simulink model "A02_L9_0"  (R2016b)
settings: Solver=ode45  StartTime=0.0  StopTime=40.0  RelTol=1e-3  EnableMultiTasking=on
settings Model: Creator=User  LastModifiedBy=mluser
settings DataIOCC: LimitDataPoints=on  SaveFormat=Array
settings OptimizationCC: LifeSpan=inf
settings DebuggingCC: SolverPrmCheckMsg=warning  SFUnexpectedBacktrackingDiag=warning  SFNoUnconditionalDefaultTransitionDiag=warning  SFExecutionAtInitializationDiag=none
settings HardwareCC: ProdBitPerPointer=32  ProdBitPerSizeT=32  ProdBitPerPtrDiffT=32  ProdLargestAtomicFloat=None  ProdIntDivRoundTo=Undefined  ProdEndianess=Unspecified  ProdWordSize=32  ProdHWDeviceType=32-bit Generic
settings ModelReferenceCC: PropagateSignalLabelsOutOfModel=off
settings GRTTargetCC: TargetLangStandard=C89/C90 (ANSI)
settings ConfigComp: CovMetricSettings=dw  CovSaveCumulativeToWorkspaceVar=on  CovSaveSingleToWorkspaceVar=on  CovExternalEMLEnable=off  CovSFcnEnable=off

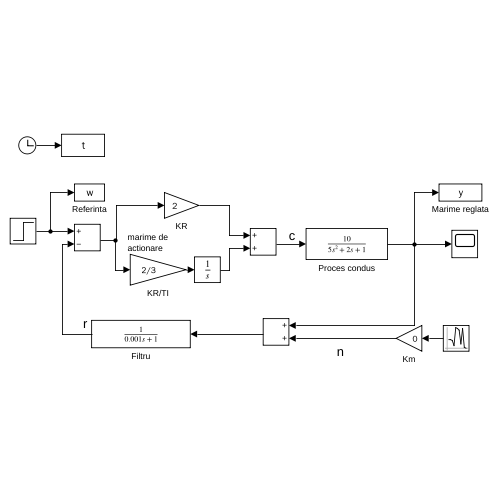
[thumbnail: Simulink's stored preview of the top-level diagram]
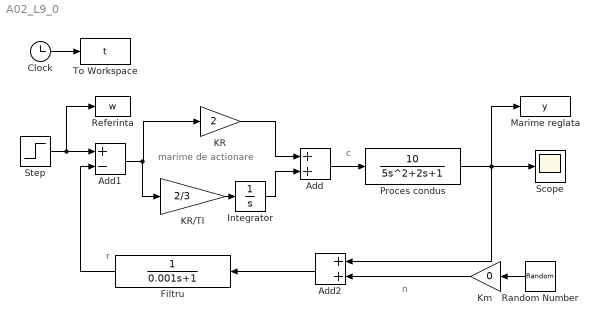
== system A02_L9_0 ==
  note: n
  note: r
  note: c
  note: marime de
      | actionare
  Add : Sum
  Add1 : Sum  Inputs=+-
  Add2 : Sum
  Clock : Clock
  Filtru : TransferFcn  Denominator=[0.001 1]
  Integrator : Integrator
  KR : Gain  Gain=2
  KR/TI : Gain  Gain=2/3
  Km : Gain  Gain=0
  Marime reglata : ToWorkspace  VariableName=y  SampleTime=-1
  Proces condus : TransferFcn  Numerator=[10]  Denominator=[5 2 1]
  Random Number : RandomNumber  SampleTime=0.1
  Referinta : ToWorkspace  VariableName=w  SampleTime=-1
  Scope : Scope
  Step : Step  Time=0  After=10  SampleTime=0
  To Workspace : ToWorkspace  VariableName=t  SampleTime=-1
  wires:
  Add/1 -> Proces condus/1
  KR/1 -> Add/1
  Integrator/1 -> Add/2
  KR/TI/1 -> Integrator/1
  Proces condus/1 -> Add2/1, Marime reglata/1, Scope/1
  Add1/1 -> KR/TI/1, KR/1
  Filtru/1 -> Add1/2
  Step/1 -> Referinta/1, Add1/1
  Add2/1 -> Filtru/1
  Random Number/1 -> Km/1
  Km/1 -> Add2/2
  Clock/1 -> To Workspace/1
